simulink model "VB_RIFKF_UWB_INS25"  (R2023a)
settings: Solver=FixedStepAuto  StartTime=0.0  StopTime=500  FixedStep=0.01  RelTol=1e-3
InitFcn:
  | resilient_initNavigation1216;
  | init_param;
  | param_bias;
undefined symbols (not defined in the file or in its folder): dt, g0, gam0_rad, ISUS_flag, lp_GPS_sample_time, lp_Lidar_knoise, lp_Lidar_max, lp_Lidar_min, lp_Lidar_sample_time, lp_Lidar_seed, lp_UWB_knoise, lp_UWB_sample_time, lp_UWB_seed, lp_UWB_XY_max, lp_UWB_XY_min, magnitude, p, P0, P0_RIEKF, param, pd0, pe0, phi0_rad, pn0, psi, psi0_rad, state_dim, vd0, ve0, vn0
libraries: simulink_extras x108, simulink x89, dspstat3 x74, sharedtransform x61, matrix_library x11, sharedTrackingLibrary x8, aerolibconvert2 x5, aerolibtransform2 x5, dspfactors x3
(part 9 of 29)

== system VB_RIFKF_UWB_INS25/No.1_Sensor_Data_Process/Magn_Data_Process ==
  magn_B_guass_ori : Inport
  Data Type Conversion : DataTypeConversion  OutDataTypeStr=single  SaturateOnIntegerOverflow=off  RndMeth=Floor
  MATLAB Function1 : MATLAB Function  Commented=on  TreatAsAtomicUnit=on
  Magn_preprocessing : Subsystem
  MAGN_Data : Outport
  wires:
  magn_B_guass_ori/1 -> Data Type Conversion/1, Magn_preprocessing/1(Magn_B_rad/s_ori)
  Data Type Conversion/1 -> MAGN_Data/1

== system VB_RIFKF_UWB_INS25/No.1_Sensor_Data_Process/Subsystem ==
  Vairspeed : Inport
  Constant : Constant  Value=0  OutDataTypeStr=single
  Mux : Mux  Inputs=3
  TD_baro : Subsystem
  Terminator : Terminator
  VairspeedData : Outport
  wires:
  TD_baro/2(H_baro_TD) -> Mux/1
  Constant/1 -> Mux/3, Mux/2
  Mux/1 -> VairspeedData/1  "VairspeedData"
  Vairspeed/1 -> TD_baro/1(H_baro)
  TD_baro/1(vH_baro_TD) -> Terminator/1  "vH_baro_m/s_TD"

== system VB_RIFKF_UWB_INS25/No.1_Sensor_Data_Process/TOF_Data_Process ==
  TOF_mm_ori : Inport
  QGC_sensor_reinit : Inport  Port=2
  Bus Creator1 : BusCreator  Inputs=4
  Data Type Conversion : DataTypeConversion  OutDataTypeStr=uint8  SaturateOnIntegerOverflow=off  RndMeth=Floor
  Data Type Conversion1 : DataTypeConversion  OutDataTypeStr=single  SaturateOnIntegerOverflow=off  RndMeth=Floor
  Demux : Demux  Outputs=3
  Gain : Gain  Gain=0.01
  Scope : Scope  NumInputPorts=2
  Scope1 : Scope  NumInputPorts=2
  Sum : Sum  Inputs=|-+
  TD_baro : Subsystem
  reinit_TOF : Subsystem
  TOF_Data : Outport
  wires:
  Sum/1 -> Data Type Conversion1/1, Scope1/2  "TOF_Dist_m"
  reinit_TOF/1(dataout) -> Sum/1, Scope1/1
  QGC_sensor_reinit/1 -> reinit_TOF/1(QGC_sensor_reinit)
  Data Type Conversion/1 -> Bus Creator1/4  "TOF_sts"
  Gain/1 -> reinit_TOF/2(Data), Sum/2  "TOF_Dist_m"
  TD_baro/1(vH_TOF_TD) -> Bus Creator1/1, Scope/1  "vH_TOF_m/s_TD"
  Bus Creator1/1 -> TOF_Data/1  "TOF_Data"
  Demux/2 -> Bus Creator1/3  "TOF_Inten"
  TOF_mm_ori/1 -> Demux/1
  Demux/1 -> Gain/1
  Demux/3 -> Data Type Conversion/1  "TOF_sts"
  TD_baro/2(H_TOF_TD) -> Scope/2, Bus Creator1/2  "H_TOF_TD"
  Data Type Conversion1/1 -> TD_baro/1(H_TOF)  "补偿姿态前"

== system VB_RIFKF_UWB_INS25/No.1_Sensor_Data_Process/baro_Data_Process ==
  baro : Inport
  QGC_sensor_reinit : Inport  Port=2
  baro_tem : Inport  Port=3
  Bus Creator : BusCreator  Inputs=2
  Constant : Constant  Value=0  OutDataTypeStr=single
  From Workspace : FromWorkspace  Commented=on  VariableName=[All.t',All.Alt_Ps]
  Gain : Gain  Gain=0.01
  Pressure2Height : Subsystem
  Scope : Scope
  Scope1 : Scope  Commented=on  NumInputPorts=2
  Sum : Sum  Inputs=|+-
  Sum1 : Sum  Commented=on  Inputs=|+-
  Sum2 : Sum  Inputs=|+-
  Switch : Switch  Criteria=u2 > Threshold  Threshold=31  SaturateOnIntegerOverflow=off  InputSameDT=off
  TD_baro : Subsystem
  TemCompensate1 : Subsystem
  reinit_baro0 : Subsystem
  reinit_baro1 : Subsystem  Commented=on
  BARO_Data : Outport  PortDimensions=2
  wires:
  baro_tem/1 -> TemCompensate1/1(baro_tem), Switch/2  "AFCbarotem"
  Pressure2Height/1(H_baro) -> TD_baro/1(H_baro)  "AFC4"
  Switch/1 -> Sum2/2
  baro/1 -> Gain/1  "AFC4"
  Constant/1 -> Switch/1
  TemCompensate1/1(bias) -> Switch/3
  Sum2/1 -> Sum/1, reinit_baro0/2(Data)
  TD_baro/2(H_baro_TD) -> Sum2/1  "H_baro_TD"
  Sum/1 -> Scope1/2, Scope/1, Bus Creator/2  "H_baro_TD"
  reinit_baro0/1(dataout) -> Sum/2
  QGC_sensor_reinit/1 -> reinit_baro1/1(QGC_sensor_reinit), reinit_baro0/1(QGC_sensor_reinit)
  Bus Creator/1 -> BARO_Data/1
  Gain/1 -> Pressure2Height/1(baro)
  TD_baro/1(vH_baro_TD) -> Bus Creator/1  "vH_baro_m/s_TD"
  From Workspace/1 -> reinit_baro1/2(Data), Sum1/1
  reinit_baro1/1(dataout) -> Sum1/2
  Sum1/1 -> Scope1/1

== system VB_RIFKF_UWB_INS25/No.1_Sensor_Data_Process1/GPS_Data_Process ==
  note: GPS_fixtype:
      | 0: 定位不可用或无效
      | 1:单点定位
      | 2:伪距差分
      | 4:RTK固定解
  GPS_Vecef_m/s : Inport
  GPS_LLA_rad : Inport  Port=2
  GPS_fixtype : Inport  Port=3
  hdop_GPS : Inport  Port=4
  QGC_sensor_reinit : Inport  Port=5
  GPS0 : Inport  Port=6
  Bus Creator : BusCreator  Inputs=13
  Demux : Demux  Outputs=3
  Demux1 : Demux  Outputs=3
  Demux3 : Demux  Outputs=3
  GPS_fixtype1 : InportShadow  Port=3
  LLA2NED : Subsystem
  heading_GPS : Subsystem
  GPS_Data : Outport
  wires:
  LLA2NED/1("gpsposNEDout ") -> Demux1/1
  GPS_fixtype1/1 -> LLA2NED/2(GPSfixtype)  "fixtype_gps"
  Bus Creator/1 -> GPS_Data/1
  Demux3/3 -> Bus Creator/3  "H_gps"
  Demux/3 -> Bus Creator/9  "vd_gps"
  Demux/1 -> Bus Creator/7  "vn_gps"
  GPS_LLA_rad/1 -> Demux3/1, LLA2NED/1(gps_LLA_rad)
  Demux/2 -> Bus Creator/8  "ve_gps"
  Demux3/2 -> Bus Creator/2  "lon_gps"
  Demux3/1 -> Bus Creator/1  "lat_gps"
  GPS_fixtype/1 -> Bus Creator/12  "fixtype_gps"
  QGC_sensor_reinit/1 -> LLA2NED/4(QGC_sensor_reinit)  "QGC_sensor_reinit"
  Demux1/1 -> Bus Creator/4  "pos_N_gps"
  Demux1/2 -> Bus Creator/5  "pos_E_gps"
  Demux1/3 -> Bus Creator/6  "pos_D_gps"
  GPS_Vecef_m/s/1 -> LLA2NED/3(GPS_Vecef_m/s)
  LLA2NED/2(gpsvNEDout) -> Demux/1, heading_GPS/1(Vned)
  heading_GPS/1(heading_GPS_rad) -> Bus Creator/10  "heading_GPS_rad"
  heading_GPS/2(heading_GPS_valid) -> Bus Creator/11  "heading_GPS_valid"
  hdop_GPS/1 -> Bus Creator/13  "hdop_GPS"
  GPS0/1 -> LLA2NED/5(GPS0)

== system VB_RIFKF_UWB_INS25/No.1_Sensor_Data_Process1/IMU_Data_Process ==
  gyro_B_rad/s_ori : Inport
  accl_B_m/s_ori : Inport  Port=2
  Bias Eliminate : Subsystem
  Bus Creator : BusCreator  Inputs=2
  accl_preprocessing2 : Subsystem  Commented=on
  gyro_preprocessing2 : Subsystem  Commented=on
  IMU_Data : Outport  PortDimensions=6
  wires:
  Bus Creator/1 -> IMU_Data/1
  accl_B_m/s_ori/1 -> Bus Creator/2  "accl_B_m/s2_LPF"
  Bias Eliminate/1(Out1) -> Bus Creator/1  "gyro_B_rad/s_LPF"
  gyro_B_rad/s_ori/1 -> Bias Eliminate/1(gyro_B_rad/s_ori)  "gyro_B_rad/s_LPF"

== system VB_RIFKF_UWB_INS25/No.1_Sensor_Data_Process1/Magn_Data_Process ==
  magn_B_guass_ori : Inport
  Data Type Conversion : DataTypeConversion  OutDataTypeStr=single  SaturateOnIntegerOverflow=off  RndMeth=Floor
  MATLAB Function1 : MATLAB Function  Commented=on  TreatAsAtomicUnit=on
  Magn_preprocessing : Subsystem
  MAGN_Data : Outport
  wires:
  Data Type Conversion/1 -> MAGN_Data/1
  magn_B_guass_ori/1 -> Magn_preprocessing/1(Magn_B_rad/s_ori), Data Type Conversion/1

== system VB_RIFKF_UWB_INS25/No.1_Sensor_Data_Process1/Subsystem ==
  Vairspeed : Inport
  Constant : Constant  Value=0  OutDataTypeStr=single
  Mux : Mux  Inputs=3
  TD_baro : Subsystem
  Terminator : Terminator
  VairspeedData : Outport
  wires:
  TD_baro/1(vH_baro_TD) -> Terminator/1  "vH_baro_m/s_TD"
  Vairspeed/1 -> TD_baro/1(H_baro)
  Mux/1 -> VairspeedData/1  "VairspeedData"
  Constant/1 -> Mux/2, Mux/3
  TD_baro/2(H_baro_TD) -> Mux/1

== system VB_RIFKF_UWB_INS25/No.1_Sensor_Data_Process1/TOF_Data_Process ==
  TOF_mm_ori : Inport
  QGC_sensor_reinit : Inport  Port=2
  Bus Creator1 : BusCreator  Inputs=4
  Data Type Conversion : DataTypeConversion  OutDataTypeStr=uint8  SaturateOnIntegerOverflow=off  RndMeth=Floor
  Data Type Conversion1 : DataTypeConversion  OutDataTypeStr=single  SaturateOnIntegerOverflow=off  RndMeth=Floor
  Demux : Demux  Outputs=3
  Gain : Gain  Gain=0.01
  Scope : Scope  NumInputPorts=2
  Scope1 : Scope  NumInputPorts=2
  Sum : Sum  Inputs=|-+
  TD_baro : Subsystem
  reinit_TOF : Subsystem
  TOF_Data : Outport
  wires:
  Data Type Conversion1/1 -> TD_baro/1(H_TOF)  "补偿姿态前"
  TD_baro/2(H_TOF_TD) -> Bus Creator1/2, Scope/2  "H_TOF_TD"
  Demux/3 -> Data Type Conversion/1  "TOF_sts"
  Demux/1 -> Gain/1
  TOF_mm_ori/1 -> Demux/1
  Demux/2 -> Bus Creator1/3  "TOF_Inten"
  Bus Creator1/1 -> TOF_Data/1  "TOF_Data"
  TD_baro/1(vH_TOF_TD) -> Scope/1, Bus Creator1/1  "vH_TOF_m/s_TD"
  Gain/1 -> Sum/2, reinit_TOF/2(Data)  "TOF_Dist_m"
  Data Type Conversion/1 -> Bus Creator1/4  "TOF_sts"
  QGC_sensor_reinit/1 -> reinit_TOF/1(QGC_sensor_reinit)
  reinit_TOF/1(dataout) -> Scope1/1, Sum/1
  Sum/1 -> Scope1/2, Data Type Conversion1/1  "TOF_Dist_m"

== system VB_RIFKF_UWB_INS25/No.1_Sensor_Data_Process1/baro_Data_Process ==
  baro : Inport
  QGC_sensor_reinit : Inport  Port=2
  baro_tem : Inport  Port=3
  Bus Creator : BusCreator  Inputs=2
  Constant : Constant  Value=0  OutDataTypeStr=single
  From Workspace : FromWorkspace  Commented=on  VariableName=[All.t',All.Alt_Ps]
  Gain : Gain  Gain=0.01
  Pressure2Height : Subsystem
  Scope : Scope
  Scope1 : Scope  Commented=on  NumInputPorts=2
  Sum : Sum  Inputs=|+-
  Sum1 : Sum  Commented=on  Inputs=|+-
  Sum2 : Sum  Inputs=|+-
  Switch : Switch  Criteria=u2 > Threshold  Threshold=31  SaturateOnIntegerOverflow=off  InputSameDT=off
  TD_baro : Subsystem
  TemCompensate1 : Subsystem
  reinit_baro0 : Subsystem
  reinit_baro1 : Subsystem  Commented=on
  BARO_Data : Outport  PortDimensions=2
  wires:
  Sum1/1 -> Scope1/1
  reinit_baro1/1(dataout) -> Sum1/2
  From Workspace/1 -> Sum1/1, reinit_baro1/2(Data)
  TD_baro/1(vH_baro_TD) -> Bus Creator/1  "vH_baro_m/s_TD"
  Gain/1 -> Pressure2Height/1(baro)
  Bus Creator/1 -> BARO_Data/1
  QGC_sensor_reinit/1 -> reinit_baro0/1(QGC_sensor_reinit), reinit_baro1/1(QGC_sensor_reinit)
  reinit_baro0/1(dataout) -> Sum/2
  Sum/1 -> Bus Creator/2, Scope/1, Scope1/2  "H_baro_TD"
  TD_baro/2(H_baro_TD) -> Sum2/1  "H_baro_TD"
  Sum2/1 -> reinit_baro0/2(Data), Sum/1
  TemCompensate1/1(bias) -> Switch/3
  Constant/1 -> Switch/1
  baro/1 -> Gain/1  "AFC4"
  Switch/1 -> Sum2/2
  Pressure2Height/1(H_baro) -> TD_baro/1(H_baro)  "AFC4"
  baro_tem/1 -> Switch/2, TemCompensate1/1(baro_tem)  "AFCbarotem"

== system VB_RIFKF_UWB_INS25/No.1_Sensor_Data_Process2/GPS_Data_Process ==
  note: GPS_fixtype:
      | 0: 定位不可用或无效
      | 1:单点定位
      | 2:伪距差分
      | 4:RTK固定解
  GPS_Vecef_m/s : Inport
  GPS_LLA_rad : Inport  Port=2
  GPS_fixtype : Inport  Port=3
  hdop_GPS : Inport  Port=4
  QGC_sensor_reinit : Inport  Port=5
  GPS0 : Inport  Port=6
  Bus Creator : BusCreator  Inputs=13
  Demux : Demux  Outputs=3
  Demux1 : Demux  Outputs=3
  Demux3 : Demux  Outputs=3
  GPS_fixtype1 : InportShadow  Port=3
  LLA2NED : Subsystem
  heading_GPS : Subsystem
  GPS_Data : Outport
  wires:
  hdop_GPS/1 -> Bus Creator/13  "hdop_GPS"
  heading_GPS/2(heading_GPS_valid) -> Bus Creator/11  "heading_GPS_valid"
  heading_GPS/1(heading_GPS_rad) -> Bus Creator/10  "heading_GPS_rad"
  LLA2NED/2(gpsvNEDout) -> heading_GPS/1(Vned), Demux/1
  GPS_Vecef_m/s/1 -> LLA2NED/3(GPS_Vecef_m/s)
  Demux1/3 -> Bus Creator/6  "pos_D_gps"
  Demux1/2 -> Bus Creator/5  "pos_E_gps"
  Demux1/1 -> Bus Creator/4  "pos_N_gps"
  QGC_sensor_reinit/1 -> LLA2NED/4(QGC_sensor_reinit)  "QGC_sensor_reinit"
  GPS_fixtype/1 -> Bus Creator/12  "fixtype_gps"
  Demux3/1 -> Bus Creator/1  "lat_gps"
  Demux3/2 -> Bus Creator/2  "lon_gps"
  Demux/2 -> Bus Creator/8  "ve_gps"
  GPS_LLA_rad/1 -> LLA2NED/1(gps_LLA_rad), Demux3/1
  Demux/1 -> Bus Creator/7  "vn_gps"
  Demux/3 -> Bus Creator/9  "vd_gps"
  Demux3/3 -> Bus Creator/3  "H_gps"
  Bus Creator/1 -> GPS_Data/1
  GPS_fixtype1/1 -> LLA2NED/2(GPSfixtype)  "fixtype_gps"
  LLA2NED/1("gpsposNEDout ") -> Demux1/1
  GPS0/1 -> LLA2NED/5(GPS0)

== system VB_RIFKF_UWB_INS25/No.1_Sensor_Data_Process2/IMU_Data_Process ==
  gyro_B_rad/s_ori : Inport
  accl_B_m/s_ori : Inport  Port=2
  Bias Eliminate : Subsystem
  Bus Creator : BusCreator  Inputs=2
  accl_preprocessing2 : Subsystem  Commented=on
  gyro_preprocessing2 : Subsystem  Commented=on
  IMU_Data : Outport  PortDimensions=6
  wires:
  gyro_B_rad/s_ori/1 -> Bias Eliminate/1(gyro_B_rad/s_ori)  "gyro_B_rad/s_LPF"
  Bias Eliminate/1(Out1) -> Bus Creator/1  "gyro_B_rad/s_LPF"
  accl_B_m/s_ori/1 -> Bus Creator/2  "accl_B_m/s2_LPF"
  Bus Creator/1 -> IMU_Data/1

== system VB_RIFKF_UWB_INS25/No.1_Sensor_Data_Process2/Magn_Data_Process ==
  magn_B_guass_ori : Inport
  Data Type Conversion : DataTypeConversion  OutDataTypeStr=single  SaturateOnIntegerOverflow=off  RndMeth=Floor
  MATLAB Function1 : MATLAB Function  Commented=on  TreatAsAtomicUnit=on
  Magn_preprocessing : Subsystem
  MAGN_Data : Outport
  wires:
  magn_B_guass_ori/1 -> Data Type Conversion/1, Magn_preprocessing/1(Magn_B_rad/s_ori)
  Data Type Conversion/1 -> MAGN_Data/1

== system VB_RIFKF_UWB_INS25/No.1_Sensor_Data_Process2/Subsystem ==
  Vairspeed : Inport
  Constant : Constant  Value=0  OutDataTypeStr=single
  Mux : Mux  Inputs=3
  TD_baro : Subsystem
  Terminator : Terminator
  VairspeedData : Outport
  wires:
  TD_baro/2(H_baro_TD) -> Mux/1
  Constant/1 -> Mux/3, Mux/2
  Mux/1 -> VairspeedData/1  "VairspeedData"
  Vairspeed/1 -> TD_baro/1(H_baro)
  TD_baro/1(vH_baro_TD) -> Terminator/1  "vH_baro_m/s_TD"

== system VB_RIFKF_UWB_INS25/No.1_Sensor_Data_Process2/TOF_Data_Process ==
  TOF_mm_ori : Inport
  QGC_sensor_reinit : Inport  Port=2
  Bus Creator1 : BusCreator  Inputs=4
  Data Type Conversion : DataTypeConversion  OutDataTypeStr=uint8  SaturateOnIntegerOverflow=off  RndMeth=Floor
  Data Type Conversion1 : DataTypeConversion  OutDataTypeStr=single  SaturateOnIntegerOverflow=off  RndMeth=Floor
  Demux : Demux  Outputs=3
  Gain : Gain  Gain=0.01
  Scope : Scope  NumInputPorts=2
  Scope1 : Scope  NumInputPorts=2
  Sum : Sum  Inputs=|-+
  TD_baro : Subsystem
  reinit_TOF : Subsystem
  TOF_Data : Outport
  wires:
  Sum/1 -> Data Type Conversion1/1, Scope1/2  "TOF_Dist_m"
  reinit_TOF/1(dataout) -> Sum/1, Scope1/1
  QGC_sensor_reinit/1 -> reinit_TOF/1(QGC_sensor_reinit)
  Data Type Conversion/1 -> Bus Creator1/4  "TOF_sts"
  Gain/1 -> reinit_TOF/2(Data), Sum/2  "TOF_Dist_m"
  TD_baro/1(vH_TOF_TD) -> Bus Creator1/1, Scope/1  "vH_TOF_m/s_TD"
  Bus Creator1/1 -> TOF_Data/1  "TOF_Data"
  Demux/2 -> Bus Creator1/3  "TOF_Inten"
  TOF_mm_ori/1 -> Demux/1
  Demux/1 -> Gain/1
  Demux/3 -> Data Type Conversion/1  "TOF_sts"
  TD_baro/2(H_TOF_TD) -> Scope/2, Bus Creator1/2  "H_TOF_TD"
  Data Type Conversion1/1 -> TD_baro/1(H_TOF)  "补偿姿态前"

== system VB_RIFKF_UWB_INS25/No.1_Sensor_Data_Process2/baro_Data_Process ==
  baro : Inport
  QGC_sensor_reinit : Inport  Port=2
  baro_tem : Inport  Port=3
  Bus Creator : BusCreator  Inputs=2
  Constant : Constant  Value=0  OutDataTypeStr=single
  From Workspace : FromWorkspace  Commented=on  VariableName=[All.t',All.Alt_Ps]
  Gain : Gain  Gain=0.01
  Pressure2Height : Subsystem
  Scope : Scope
  Scope1 : Scope  Commented=on  NumInputPorts=2
  Sum : Sum  Inputs=|+-
  Sum1 : Sum  Commented=on  Inputs=|+-
  Sum2 : Sum  Inputs=|+-
  Switch : Switch  Criteria=u2 > Threshold  Threshold=31  SaturateOnIntegerOverflow=off  InputSameDT=off
  TD_baro : Subsystem
  TemCompensate1 : Subsystem
  reinit_baro0 : Subsystem
  reinit_baro1 : Subsystem  Commented=on
  BARO_Data : Outport  PortDimensions=2
  wires:
  baro_tem/1 -> TemCompensate1/1(baro_tem), Switch/2  "AFCbarotem"
  Pressure2Height/1(H_baro) -> TD_baro/1(H_baro)  "AFC4"
  Switch/1 -> Sum2/2
  baro/1 -> Gain/1  "AFC4"
  Constant/1 -> Switch/1
  TemCompensate1/1(bias) -> Switch/3
  Sum2/1 -> Sum/1, reinit_baro0/2(Data)
  TD_baro/2(H_baro_TD) -> Sum2/1  "H_baro_TD"
  Sum/1 -> Scope1/2, Scope/1, Bus Creator/2  "H_baro_TD"
  reinit_baro0/1(dataout) -> Sum/2
  QGC_sensor_reinit/1 -> reinit_baro1/1(QGC_sensor_reinit), reinit_baro0/1(QGC_sensor_reinit)
  Bus Creator/1 -> BARO_Data/1
  Gain/1 -> Pressure2Height/1(baro)
  TD_baro/1(vH_baro_TD) -> Bus Creator/1  "vH_baro_m/s_TD"
  From Workspace/1 -> reinit_baro1/2(Data), Sum1/1
  reinit_baro1/1(dataout) -> Sum1/2
  Sum1/1 -> Scope1/1

== system VB_RIFKF_UWB_INS25/No.1_Sensor_Data_Process3/GPS_Data_Process ==
  note: GPS_fixtype:
      | 0: 定位不可用或无效
      | 1:单点定位
      | 2:伪距差分
      | 4:RTK固定解
  GPS_Vecef_m/s : Inport
  GPS_LLA_rad : Inport  Port=2
  GPS_fixtype : Inport  Port=3
  hdop_GPS : Inport  Port=4
  QGC_sensor_reinit : Inport  Port=5
  Bus Creator : BusCreator  Inputs=13
  Demux : Demux  Outputs=3
  Demux1 : Demux  Outputs=3
  Demux3 : Demux  Outputs=3
  GPS_fixtype1 : InportShadow  Port=3
  LLA2NED : Subsystem
  heading_GPS : Subsystem
  GPS_Data : Outport
  wires:
  LLA2NED/1("gpsposNEDout ") -> Demux1/1
  GPS_fixtype1/1 -> LLA2NED/2(GPSfixtype)  "fixtype_gps"
  Bus Creator/1 -> GPS_Data/1
  Demux3/3 -> Bus Creator/3  "H_gps"
  Demux/3 -> Bus Creator/9  "vd_gps"
  Demux/1 -> Bus Creator/7  "vn_gps"
  GPS_LLA_rad/1 -> Demux3/1, LLA2NED/1(gps_LLA_rad)
  Demux/2 -> Bus Creator/8  "ve_gps"
  Demux3/2 -> Bus Creator/2  "lon_gps"
  Demux3/1 -> Bus Creator/1  "lat_gps"
  GPS_fixtype/1 -> Bus Creator/12  "fixtype_gps"
  QGC_sensor_reinit/1 -> LLA2NED/4(QGC_sensor_reinit)  "QGC_sensor_reinit"
  Demux1/1 -> Bus Creator/4  "pos_N_gps"
  Demux1/2 -> Bus Creator/5  "pos_E_gps"
  Demux1/3 -> Bus Creator/6  "pos_D_gps"
  GPS_Vecef_m/s/1 -> LLA2NED/3(GPS_Vecef_m/s)
  LLA2NED/2(gpsvNEDout) -> Demux/1, heading_GPS/1(Vned)
  heading_GPS/1(heading_GPS_rad) -> Bus Creator/10  "heading_GPS_rad"
  heading_GPS/2(heading_GPS_valid) -> Bus Creator/11  "heading_GPS_valid"
  hdop_GPS/1 -> Bus Creator/13  "hdop_GPS"

== system VB_RIFKF_UWB_INS25/No.1_Sensor_Data_Process3/IMU_Data_Process ==
  gyro_B_rad/s_ori : Inport
  accl_B_m/s_ori : Inport  Port=2
  Bias Eliminate : Subsystem
  Bus Creator : BusCreator  Inputs=2
  accl_preprocessing2 : Subsystem  Commented=on
  gyro_preprocessing2 : Subsystem  Commented=on
  IMU_Data : Outport  PortDimensions=6
  wires:
  Bus Creator/1 -> IMU_Data/1
  accl_B_m/s_ori/1 -> Bus Creator/2  "accl_B_m/s2_LPF"
  Bias Eliminate/1(Out1) -> Bus Creator/1  "gyro_B_rad/s_LPF"
  gyro_B_rad/s_ori/1 -> Bias Eliminate/1(gyro_B_rad/s_ori)  "gyro_B_rad/s_LPF"

== system VB_RIFKF_UWB_INS25/No.1_Sensor_Data_Process3/Magn_Data_Process ==
  magn_B_guass_ori : Inport
  Data Type Conversion : DataTypeConversion  OutDataTypeStr=single  SaturateOnIntegerOverflow=off  RndMeth=Floor
  MATLAB Function1 : MATLAB Function  Commented=on  TreatAsAtomicUnit=on
  Magn_preprocessing : Subsystem
  MAGN_Data : Outport
  wires:
  Data Type Conversion/1 -> MAGN_Data/1
  magn_B_guass_ori/1 -> Magn_preprocessing/1(Magn_B_rad/s_ori), Data Type Conversion/1

== system VB_RIFKF_UWB_INS25/No.1_Sensor_Data_Process3/Subsystem ==
  Vairspeed : Inport
  Constant : Constant  Value=0  OutDataTypeStr=single
  Mux : Mux  Inputs=3
  TD_baro : Subsystem
  Terminator : Terminator
  VairspeedData : Outport
  wires:
  TD_baro/1(vH_baro_TD) -> Terminator/1  "vH_baro_m/s_TD"
  Vairspeed/1 -> TD_baro/1(H_baro)
  Mux/1 -> VairspeedData/1  "VairspeedData"
  Constant/1 -> Mux/2, Mux/3
  TD_baro/2(H_baro_TD) -> Mux/1

== system VB_RIFKF_UWB_INS25/No.1_Sensor_Data_Process3/TOF_Data_Process ==
  TOF_mm_ori : Inport
  QGC_sensor_reinit : Inport  Port=2
  Bus Creator1 : BusCreator  Inputs=4
  Data Type Conversion : DataTypeConversion  OutDataTypeStr=uint8  SaturateOnIntegerOverflow=off  RndMeth=Floor
  Data Type Conversion1 : DataTypeConversion  OutDataTypeStr=single  SaturateOnIntegerOverflow=off  RndMeth=Floor
  Demux : Demux  Outputs=3
  Gain : Gain  Gain=0.01
  Scope : Scope  NumInputPorts=2
  Scope1 : Scope  NumInputPorts=2
  Sum : Sum  Inputs=|-+
  TD_baro : Subsystem
  reinit_TOF : Subsystem
  TOF_Data : Outport
  wires:
  Data Type Conversion1/1 -> TD_baro/1(H_TOF)  "补偿姿态前"
  TD_baro/2(H_TOF_TD) -> Bus Creator1/2, Scope/2  "H_TOF_TD"
  Demux/3 -> Data Type Conversion/1  "TOF_sts"
  Demux/1 -> Gain/1
  TOF_mm_ori/1 -> Demux/1
  Demux/2 -> Bus Creator1/3  "TOF_Inten"
  Bus Creator1/1 -> TOF_Data/1  "TOF_Data"
  TD_baro/1(vH_TOF_TD) -> Scope/1, Bus Creator1/1  "vH_TOF_m/s_TD"
  Gain/1 -> Sum/2, reinit_TOF/2(Data)  "TOF_Dist_m"
  Data Type Conversion/1 -> Bus Creator1/4  "TOF_sts"
  QGC_sensor_reinit/1 -> reinit_TOF/1(QGC_sensor_reinit)
  reinit_TOF/1(dataout) -> Scope1/1, Sum/1
  Sum/1 -> Scope1/2, Data Type Conversion1/1  "TOF_Dist_m"

== system VB_RIFKF_UWB_INS25/No.1_Sensor_Data_Process3/baro_Data_Process ==
  baro : Inport
  QGC_sensor_reinit : Inport  Port=2
  baro_tem : Inport  Port=3
  Bus Creator : BusCreator  Inputs=2
  Constant : Constant  Value=0  OutDataTypeStr=single
  From Workspace : FromWorkspace  Commented=on  VariableName=[All.t',All.Alt_Ps]
  Gain : Gain  Gain=0.01
  Pressure2Height : Subsystem
  Scope : Scope
  Scope1 : Scope  Commented=on  NumInputPorts=2
  Sum : Sum  Inputs=|+-
  Sum1 : Sum  Commented=on  Inputs=|+-
  Sum2 : Sum  Inputs=|+-
  Switch : Switch  Criteria=u2 > Threshold  Threshold=31  SaturateOnIntegerOverflow=off  InputSameDT=off
  TD_baro : Subsystem
  TemCompensate1 : Subsystem
  reinit_baro0 : Subsystem
  reinit_baro1 : Subsystem  Commented=on
  BARO_Data : Outport  PortDimensions=2
  wires:
  Sum1/1 -> Scope1/1
  reinit_baro1/1(dataout) -> Sum1/2
  From Workspace/1 -> Sum1/1, reinit_baro1/2(Data)
  TD_baro/1(vH_baro_TD) -> Bus Creator/1  "vH_baro_m/s_TD"
  Gain/1 -> Pressure2Height/1(baro)
  Bus Creator/1 -> BARO_Data/1
  QGC_sensor_reinit/1 -> reinit_baro0/1(QGC_sensor_reinit), reinit_baro1/1(QGC_sensor_reinit)
  reinit_baro0/1(dataout) -> Sum/2
  Sum/1 -> Bus Creator/2, Scope/1, Scope1/2  "H_baro_TD"
  TD_baro/2(H_baro_TD) -> Sum2/1  "H_baro_TD"
  Sum2/1 -> reinit_baro0/2(Data), Sum/1
  TemCompensate1/1(bias) -> Switch/3
  Constant/1 -> Switch/1
  baro/1 -> Gain/1  "AFC4"
  Switch/1 -> Sum2/2
  Pressure2Height/1(H_baro) -> TD_baro/1(H_baro)  "AFC4"
  baro_tem/1 -> Switch/2, TemCompensate1/1(baro_tem)  "AFCbarotem"

== system VB_RIFKF_UWB_INS25/No.1_Sensor_Data_Process4/GPS_Data_Process ==
  note: GPS_fixtype:
      | 0: 定位不可用或无效
      | 1:单点定位
      | 2:伪距差分
      | 4:RTK固定解
  GPS_Vecef_m/s : Inport
  GPS_LLA_rad : Inport  Port=2
  GPS_fixtype : Inport  Port=3
  hdop_GPS : Inport  Port=4
  QGC_sensor_reinit : Inport  Port=5
  Bus Creator : BusCreator  Inputs=13
  Demux : Demux  Outputs=3
  Demux1 : Demux  Outputs=3
  Demux3 : Demux  Outputs=3
  GPS_fixtype1 : InportShadow  Port=3
  LLA2NED : Subsystem
  heading_GPS : Subsystem
  GPS_Data : Outport
  GPS0 : Outport  Port=2
  GPS_noerr : Outport  Port=3
  wires:
  LLA2NED/4(gpsposNED_noerr) -> GPS_noerr/1
  LLA2NED/3(GPS0) -> GPS0/1
  LLA2NED/1("gpsposNEDout ") -> Demux1/1
  GPS_fixtype1/1 -> LLA2NED/2(GPSfixtype)  "fixtype_gps"
  Bus Creator/1 -> GPS_Data/1
  Demux3/3 -> Bus Creator/3  "H_gps"
  Demux/3 -> Bus Creator/9  "vd_gps"
  Demux/1 -> Bus Creator/7  "vn_gps"
  GPS_LLA_rad/1 -> Demux3/1, LLA2NED/1(gps_LLA_rad)
  Demux/2 -> Bus Creator/8  "ve_gps"
  Demux3/2 -> Bus Creator/2  "lon_gps"
  Demux3/1 -> Bus Creator/1  "lat_gps"
  GPS_fixtype/1 -> Bus Creator/12  "fixtype_gps"
  QGC_sensor_reinit/1 -> LLA2NED/4(QGC_sensor_reinit)  "QGC_sensor_reinit"
  Demux1/1 -> Bus Creator/4  "pos_N_gps"
  Demux1/2 -> Bus Creator/5  "pos_E_gps"
  Demux1/3 -> Bus Creator/6  "pos_D_gps"
  GPS_Vecef_m/s/1 -> LLA2NED/3(GPS_Vecef_m/s)
  LLA2NED/2(gpsvNEDout) -> Demux/1, heading_GPS/1(Vned)
  heading_GPS/1(heading_GPS_rad) -> Bus Creator/10  "heading_GPS_rad"
  heading_GPS/2(heading_GPS_valid) -> Bus Creator/11  "heading_GPS_valid"
  hdop_GPS/1 -> Bus Creator/13  "hdop_GPS"

== system VB_RIFKF_UWB_INS25/No.1_Sensor_Data_Process4/IMU_Data_Process ==
  gyro_B_rad/s_ori : Inport
  accl_B_m/s_ori : Inport  Port=2
  Bias Eliminate : Subsystem
  Bus Creator : BusCreator  Inputs=2
  accl_preprocessing2 : Subsystem  Commented=on
  gyro_preprocessing2 : Subsystem  Commented=on
  IMU_Data : Outport  PortDimensions=6
  wires:
  Bus Creator/1 -> IMU_Data/1
  accl_B_m/s_ori/1 -> Bus Creator/2  "accl_B_m/s2_LPF"
  Bias Eliminate/1(Out1) -> Bus Creator/1  "gyro_B_rad/s_LPF"
  gyro_B_rad/s_ori/1 -> Bias Eliminate/1(gyro_B_rad/s_ori)  "gyro_B_rad/s_LPF"

== system VB_RIFKF_UWB_INS25/No.1_Sensor_Data_Process4/Magn_Data_Process ==
  magn_B_guass_ori : Inport
  Data Type Conversion : DataTypeConversion  OutDataTypeStr=single  SaturateOnIntegerOverflow=off  RndMeth=Floor
  MATLAB Function1 : MATLAB Function  Commented=on  TreatAsAtomicUnit=on
  Magn_preprocessing : Subsystem
  MAGN_Data : Outport
  wires:
  Data Type Conversion/1 -> MAGN_Data/1
  magn_B_guass_ori/1 -> Magn_preprocessing/1(Magn_B_rad/s_ori), Data Type Conversion/1

== system VB_RIFKF_UWB_INS25/No.1_Sensor_Data_Process4/Subsystem ==
  Vairspeed : Inport
  Constant : Constant  Value=0  OutDataTypeStr=single
  Mux : Mux  Inputs=3
  TD_baro : Subsystem
  Terminator : Terminator
  VairspeedData : Outport
  wires:
  TD_baro/1(vH_baro_TD) -> Terminator/1  "vH_baro_m/s_TD"
  Vairspeed/1 -> TD_baro/1(H_baro)
  Mux/1 -> VairspeedData/1  "VairspeedData"
  Constant/1 -> Mux/2, Mux/3
  TD_baro/2(H_baro_TD) -> Mux/1

== system VB_RIFKF_UWB_INS25/No.1_Sensor_Data_Process4/TOF_Data_Process ==
  TOF_mm_ori : Inport
  QGC_sensor_reinit : Inport  Port=2
  Bus Creator1 : BusCreator  Inputs=4
  Data Type Conversion : DataTypeConversion  OutDataTypeStr=uint8  SaturateOnIntegerOverflow=off  RndMeth=Floor
  Data Type Conversion1 : DataTypeConversion  OutDataTypeStr=single  SaturateOnIntegerOverflow=off  RndMeth=Floor
  Demux : Demux  Outputs=3
  Gain : Gain  Gain=0.01
  Scope : Scope  NumInputPorts=2
  Scope1 : Scope  NumInputPorts=2
  Sum : Sum  Inputs=|-+
  TD_baro : Subsystem
  reinit_TOF : Subsystem
  TOF_Data : Outport
  wires:
  Data Type Conversion1/1 -> TD_baro/1(H_TOF)  "补偿姿态前"
  TD_baro/2(H_TOF_TD) -> Bus Creator1/2, Scope/2  "H_TOF_TD"
  Demux/3 -> Data Type Conversion/1  "TOF_sts"
  Demux/1 -> Gain/1
  TOF_mm_ori/1 -> Demux/1
  Demux/2 -> Bus Creator1/3  "TOF_Inten"
  Bus Creator1/1 -> TOF_Data/1  "TOF_Data"
  TD_baro/1(vH_TOF_TD) -> Scope/1, Bus Creator1/1  "vH_TOF_m/s_TD"
  Gain/1 -> Sum/2, reinit_TOF/2(Data)  "TOF_Dist_m"
  Data Type Conversion/1 -> Bus Creator1/4  "TOF_sts"
  QGC_sensor_reinit/1 -> reinit_TOF/1(QGC_sensor_reinit)
  reinit_TOF/1(dataout) -> Scope1/1, Sum/1
  Sum/1 -> Scope1/2, Data Type Conversion1/1  "TOF_Dist_m"

== system VB_RIFKF_UWB_INS25/No.1_Sensor_Data_Process4/baro_Data_Process ==
  baro : Inport
  QGC_sensor_reinit : Inport  Port=2
  baro_tem : Inport  Port=3
  Bus Creator : BusCreator  Inputs=2
  Constant : Constant  Value=0  OutDataTypeStr=single
  From Workspace : FromWorkspace  Commented=on  VariableName=[All.t',All.Alt_Ps]
  Gain : Gain  Gain=0.01
  Pressure2Height : Subsystem
  Scope : Scope
  Scope1 : Scope  Commented=on  NumInputPorts=2
  Sum : Sum  Inputs=|+-
  Sum1 : Sum  Commented=on  Inputs=|+-
  Sum2 : Sum  Inputs=|+-
  Switch : Switch  Criteria=u2 > Threshold  Threshold=31  SaturateOnIntegerOverflow=off  InputSameDT=off
  TD_baro : Subsystem
  TemCompensate1 : Subsystem
  reinit_baro0 : Subsystem
  reinit_baro1 : Subsystem  Commented=on
  BARO_Data : Outport  PortDimensions=2
  wires:
  Sum1/1 -> Scope1/1
  reinit_baro1/1(dataout) -> Sum1/2
  From Workspace/1 -> Sum1/1, reinit_baro1/2(Data)
  TD_baro/1(vH_baro_TD) -> Bus Creator/1  "vH_baro_m/s_TD"
  Gain/1 -> Pressure2Height/1(baro)
  Bus Creator/1 -> BARO_Data/1
  QGC_sensor_reinit/1 -> reinit_baro0/1(QGC_sensor_reinit), reinit_baro1/1(QGC_sensor_reinit)
  reinit_baro0/1(dataout) -> Sum/2
  Sum/1 -> Bus Creator/2, Scope/1, Scope1/2  "H_baro_TD"
  TD_baro/2(H_baro_TD) -> Sum2/1  "H_baro_TD"
  Sum2/1 -> reinit_baro0/2(Data), Sum/1
  TemCompensate1/1(bias) -> Switch/3
  Constant/1 -> Switch/1
  baro/1 -> Gain/1  "AFC4"
  Switch/1 -> Sum2/2
  Pressure2Height/1(H_baro) -> TD_baro/1(H_baro)  "AFC4"
  baro_tem/1 -> Switch/2, TemCompensate1/1(baro_tem)  "AFCbarotem"

== system VB_RIFKF_UWB_INS25/read FC1_hf/Subsystem ==
  u : Inport
  MATLAB Function : MATLAB Function  TreatAsAtomicUnit=on
  Memory : Memory
  y : Outport
  wires:
  Memory/1 -> MATLAB Function/2(u_1)
  MATLAB Function/1(y) -> y/1, Memory/1
  u/1 -> MATLAB Function/1(u)

== system VB_RIFKF_UWB_INS25/read FC1_hf/Subsystem1 ==
  u : Inport
  MATLAB Function : MATLAB Function  TreatAsAtomicUnit=on
  Memory : Memory
  y : Outport
  wires:
  u/1 -> MATLAB Function/1(u)
  MATLAB Function/1(y) -> Memory/1, y/1
  Memory/1 -> MATLAB Function/2(u_1)

== system VB_RIFKF_UWB_INS25/read FC1_hf/Subsystem2 ==
  u : Inport
  MATLAB Function : MATLAB Function  TreatAsAtomicUnit=on
  Memory : Memory
  y : Outport
  wires:
  Memory/1 -> MATLAB Function/2(u_1)
  MATLAB Function/1(y) -> y/1, Memory/1
  u/1 -> MATLAB Function/1(u)

== system VB_RIFKF_UWB_INS25/read FC1_hf/Subsystem3 ==
  u : Inport
  MATLAB Function : MATLAB Function  TreatAsAtomicUnit=on
  Memory : Memory
  y : Outport
  wires:
  u/1 -> MATLAB Function/1(u)
  MATLAB Function/1(y) -> Memory/1, y/1
  Memory/1 -> MATLAB Function/2(u_1)

== system VB_RIFKF_UWB_INS25/read FC1_hf/Subsystem4 ==
  u : Inport
  MATLAB Function : MATLAB Function  TreatAsAtomicUnit=on
  Memory : Memory
  y : Outport
  wires:
  Memory/1 -> MATLAB Function/2(u_1)
  MATLAB Function/1(y) -> y/1, Memory/1
  u/1 -> MATLAB Function/1(u)

== system VB_RIFKF_UWB_INS25/read FC1_hf/Subsystem5 ==
  u : Inport
  MATLAB Function : MATLAB Function  TreatAsAtomicUnit=on
  Memory : Memory
  y : Outport
  wires:
  u/1 -> MATLAB Function/1(u)
  MATLAB Function/1(y) -> Memory/1, y/1
  Memory/1 -> MATLAB Function/2(u_1)

== system VB_RIFKF_UWB_INS25/read FC1_hf/Subsystem6 ==
  u : Inport
  MATLAB Function : MATLAB Function  TreatAsAtomicUnit=on
  Memory : Memory
  y : Outport
  wires:
  Memory/1 -> MATLAB Function/2(u_1)
  MATLAB Function/1(y) -> y/1, Memory/1
  u/1 -> MATLAB Function/1(u)

== system VB_RIFKF_UWB_INS25/read FC1_hf/Subsystem7 ==
  u : Inport
  MATLAB Function : MATLAB Function  TreatAsAtomicUnit=on
  Memory : Memory
  y : Outport
  wires:
  u/1 -> MATLAB Function/1(u)
  MATLAB Function/1(y) -> Memory/1, y/1
  Memory/1 -> MATLAB Function/2(u_1)

== system VB_RIFKF_UWB_INS25/read FC1_hf/Subsystem8 ==
  u : Inport
  MATLAB Function : MATLAB Function  TreatAsAtomicUnit=on
  Memory : Memory
  y : Outport
  wires:
  Memory/1 -> MATLAB Function/2(u_1)
  MATLAB Function/1(y) -> y/1, Memory/1
  u/1 -> MATLAB Function/1(u)

== system VB_RIFKF_UWB_INS25/read FC1_zy/Subsystem ==
  u : Inport
  MATLAB Function : MATLAB Function  TreatAsAtomicUnit=on
  Memory : Memory
  y : Outport
  wires:
  Memory/1 -> MATLAB Function/2(u_1)
  MATLAB Function/1(y) -> y/1, Memory/1
  u/1 -> MATLAB Function/1(u)

== system VB_RIFKF_UWB_INS25/read FC1_zy/Subsystem1 ==
  u : Inport
  MATLAB Function : MATLAB Function  TreatAsAtomicUnit=on
  Memory : Memory
  y : Outport
  wires:
  u/1 -> MATLAB Function/1(u)
  MATLAB Function/1(y) -> Memory/1, y/1
  Memory/1 -> MATLAB Function/2(u_1)

== system VB_RIFKF_UWB_INS25/read FC1_zy/Subsystem2 ==
  u : Inport
  MATLAB Function : MATLAB Function  TreatAsAtomicUnit=on
  Memory : Memory
  y : Outport
  wires:
  Memory/1 -> MATLAB Function/2(u_1)
  MATLAB Function/1(y) -> y/1, Memory/1
  u/1 -> MATLAB Function/1(u)

== system VB_RIFKF_UWB_INS25/read FC6_zy2/Subsystem ==
  u : Inport
  MATLAB Function : MATLAB Function  TreatAsAtomicUnit=on
  Memory : Memory
  y : Outport
  wires:
  Memory/1 -> MATLAB Function/2(u_1)
  MATLAB Function/1(y) -> y/1, Memory/1
  u/1 -> MATLAB Function/1(u)

== system VB_RIFKF_UWB_INS25/read FC6_zy2/Subsystem1 ==
  u : Inport
  MATLAB Function : MATLAB Function  TreatAsAtomicUnit=on
  Memory : Memory
  y : Outport
  wires:
  u/1 -> MATLAB Function/1(u)
  MATLAB Function/1(y) -> Memory/1, y/1
  Memory/1 -> MATLAB Function/2(u_1)

== system VB_RIFKF_UWB_INS25/read FC6_zy2/Subsystem2 ==
  u : Inport
  MATLAB Function : MATLAB Function  TreatAsAtomicUnit=on
  Memory : Memory
  y : Outport
  wires:
  Memory/1 -> MATLAB Function/2(u_1)
  MATLAB Function/1(y) -> y/1, Memory/1
  u/1 -> MATLAB Function/1(u)

== system VB_RIFKF_UWB_INS25/相对传感器模拟1/Subsystem ==
  "psi " : Inport
  laser model : Subsystem
  psi  out : Outport
  wires:
  "psi "/1 -> laser model/1(psi & theta)
  laser model/1(psi out) -> psi  out/1

== system VB_RIFKF_UWB_INS25/相对传感器模拟1/Subsystem2 ==
  r_xyz : Inport
  radar model : Subsystem
  r_xyz out : Outport
  wires:
  r_xyz/1 -> radar model/1(r_xyz)
  radar model/1(r_xyz out) -> r_xyz out/1

== system VB_RIFKF_UWB_INS25/相对传感器模拟2/Subsystem ==
  "psi " : Inport
  laser model : Subsystem
  psi  out : Outport
  wires:
  laser model/1(psi out) -> psi  out/1
  "psi "/1 -> laser model/1(psi & theta)

== system VB_RIFKF_UWB_INS25/相对传感器模拟2/Subsystem2 ==
  r_xyz : Inport
  radar model : Subsystem
  r_xyz out : Outport
  wires:
  radar model/1(r_xyz out) -> r_xyz out/1
  r_xyz/1 -> radar model/1(r_xyz)

== system VB_RIFKF_UWB_INS25/相对传感器模拟3/Subsystem ==
  "psi " : Inport
  laser model : Subsystem
  psi  out : Outport
  wires:
  laser model/1(psi out) -> psi  out/1
  "psi "/1 -> laser model/1(psi & theta)

== system VB_RIFKF_UWB_INS25/相对传感器模拟3/Subsystem2 ==
  r_xyz : Inport
  radar model : Subsystem
  r_xyz out : Outport
  wires:
  radar model/1(r_xyz out) -> r_xyz out/1
  r_xyz/1 -> radar model/1(r_xyz)

== system VB_RIFKF_UWB_INS25/相对传感器模拟4/Subsystem ==
  "psi " : Inport
  laser model : Subsystem
  psi  out : Outport
  wires:
  "psi "/1 -> laser model/1(psi & theta)
  laser model/1(psi out) -> psi  out/1

== system VB_RIFKF_UWB_INS25/相对传感器模拟4/Subsystem2 ==
  r_xyz : Inport
  radar model : Subsystem
  r_xyz out : Outport
  wires:
  r_xyz/1 -> radar model/1(r_xyz)
  radar model/1(r_xyz out) -> r_xyz out/1

== system VB_RIFKF_UWB_INS25/ER EKF M1/Bus_Constructor2/Rotation_output ==
  RotationData : Inport
  Bus Creator : BusCreator  Inputs=4
  Bus Selector3 : BusSelector  OutputSignals=DCM_b_n
  Data Type Conversion1 : DataTypeConversion  OutDataTypeStr=single  SaturateOnIntegerOverflow=off  RndMeth=Floor
  Data Type Conversion11 : DataTypeConversion  OutDataTypeStr=single  SaturateOnIntegerOverflow=off  RndMeth=Floor
  Data Type Conversion12 : DataTypeConversion  OutDataTypeStr=double  SaturateOnIntegerOverflow=off  RndMeth=Floor
  Demux : Demux  Outputs=3
  Direction Cosine Matrix to Rotation Angles : sharedtransform/Direction Cosine Matrix to Rotation Angles  rotationOrder=ZYX  aMode=aMode  action=None  tolerance=eps(2)
      settings: LibrarySourceBlock=|
      | aerolibtransform2/Direction Cosine Matrix
      | to Rotation Angles
  Direction Cosine Matrix to Quaternions : sharedtransform/Direction Cosine Matrix  to Quaternions  aMode=0  action=None  tolerance=eps(2)
      settings: LibrarySourceBlock=|
      | aerolibtransform2/Direction Cosine Matrix
      | to Quaternions
  Radians to Degrees : simulink_extras/Transformations/Radians to Degrees
  Scope : Scope
  Signal Copy1 : SignalConversion  OverrideOpt=off
  Transpose : Math  Operator=transpose
  psi_theta_phi_rad : Outport
  wires:
  Direction Cosine Matrix to Quaternions/1 -> Data Type Conversion1/1  "q"
  Radians to Degrees/1 -> Data Type Conversion11/1
  Transpose/1 -> Data Type Conversion12/1
  Data Type Conversion12/1 -> Direction Cosine Matrix to Quaternions/1, Direction Cosine Matrix to Rotation Angles/1
  RotationData/1 -> Signal Copy1/1
  Signal Copy1/1 -> Bus Selector3/1
  Bus Selector3/1 -> Transpose/1  "<DCM_b_n>"
  Direction Cosine Matrix to Rotation Angles/1 -> Radians to Degrees/1  "psi_theta_phi"
  Bus Creator/1 -> psi_theta_phi_rad/1
  Demux/1 -> Bus Creator/1  "psi_rad"
  Demux/2 -> Bus Creator/2  "theta_rad"
  Demux/3 -> Bus Creator/3  "phi_rad"
  Data Type Conversion11/1 -> Scope/1, Demux/1  "ER EKF"
  Data Type Conversion1/1 -> Bus Creator/4  "q"

== system VB_RIFKF_UWB_INS25/ER EKF M1/Error State Kalman Filter/Cal Q1 ==
  Constant : Constant  Value=dt  OutDataTypeStr=double
  MATLAB Function1 : MATLAB Function  TreatAsAtomicUnit=on
  Qd : Outport
  wires:
  MATLAB Function1/1(Q) -> Qd/1
  Constant/1 -> MATLAB Function1/1(dt)

== system VB_RIFKF_UWB_INS25/ER EKF M1/Error State Kalman Filter/Extended Kalman Filter1 ==
  Q : Inport
  Enable1 : Inport  Port=2
  y1 : Inport  Port=3
  R1 : Inport  Port=4
  BlockOrdering : Constant  Value=true()  OutDataTypeStr=boolean
  Correct1 : Subsystem  AncestorBlock=sharedTrackingLibrary/Extras/EKFCorrect  TreatAsAtomicUnit=on  SystemSampleTime=p.SampleTimes.MeasurementFcn(1)  mask(EKFCorrect){ProcessedMaskData=p}
      mask init:
      | if strcmp(get_param(bdroot,'SimulationStatus'),'stopped')
      |     pM = [];
      |     SampleTime = [];
      |     DataType = [];
      |     SLFcnsToRegister = {};
      | else
      |     [pM,SampleTime] = ...
      |         matlabshared.tracking.internal.blocks.maskInitializationFcnEKFCorrector...
      |         (gcbh, ProcessedMaskData);
      |     [DataType,SLFcnsToRegister] = ...
      |         matlabshared.tracking.internal.blocks.maskInitializationFcnRegisterSLFcn(ProcessedMaskData, pM);
      | end
      settings: LibrarySourceBlock=sharedTrackingLibrary/Extras/EKFCorrect
  DataStoreMemory - P : DataStoreMemory  DataStoreName=P  InitialValue=p.InitialCovariance  ShowAdditionalParam=off  OutDataTypeStr=p.DataType
  DataStoreMemory - x : DataStoreMemory  DataStoreName=x  InitialValue=p.InitialState  ShowAdditionalParam=off  OutDataTypeStr=p.DataType
  DataTypeConversion_Enable1 : DataTypeConversion  OutDataTypeStr=boolean  SaturateOnIntegerOverflow=off  RndMeth=Floor
  DataTypeConversion_Q : DataTypeConversion  OutDataTypeStr=p.DataType  SaturateOnIntegerOverflow=off  RndMeth=Floor
  DataTypeConversion_R1 : DataTypeConversion  OutDataTypeStr=p.DataType  SaturateOnIntegerOverflow=off  RndMeth=Floor
  DataTypeConversion_uMeas1 : DataTypeConversion  OutDataTypeStr=p.DataType  SaturateOnIntegerOverflow=off  RndMeth=Floor
  DataTypeConversion_uState : DataTypeConversion  OutDataTypeStr=p.DataType  SaturateOnIntegerOverflow=off  RndMeth=Floor
  DataTypeConversion_y1 : DataTypeConversion  OutDataTypeStr=p.DataType  SaturateOnIntegerOverflow=off  RndMeth=Floor
  MeasurementFcn1Inputs : Constant  Value=0  OutDataTypeStr=p.DataType  SampleTime=p.SampleTimes.MeasurementFcn(1)
  Output : Subsystem  TreatAsAtomicUnit=on  SystemSampleTime=p.SampleTimes.Output
  Predict : Subsystem  TreatAsAtomicUnit=on  SystemSampleTime=p.SampleTimes.StateTransitionFcn  mask(EKFPredict){ProcessedMaskData=p}
      mask init:
      | if strcmp(get_param(bdroot,'SimulationStatus'),'stopped')
      |     pS = [];
      |     SampleTime = [];
      |     DataType = [];
      |     SLFcnsToRegister = {};
      | else
      |     [pS,SampleTime] = ...
      |         matlabshared.tracking.internal.blocks.maskInitializationFcnEKFPredictor(ProcessedMaskData);
      |     [DataType,SLFcnsToRegister] = ...
      |         matlabshared.tracking.internal.blocks.maskInitializationFcnRegisterSLFcn(ProcessedMaskData, pS);
      | end
  StateTransitionFcnInputs : Constant  Value=0  OutDataTypeStr=p.DataType  SampleTime=p.SampleTimes.StateTransitionFcn
  checkMeasurementFcn1Signals : S-Function  FunctionName=ekfukfCheckSignals  Parameters=signalCheck.BlockPath, signalCheck.MeasurementFcn{1}.PortNames, signalCheck.MeasurementFcn{1}.SampleTime, signalCheck.DataType, signalCheck.MeasurementFcn{1}.PortDimensions, 1, signalCheck.MeasurementFcn{1}.HasAdditiveNoise  SFunctionDeploymentMode=off  EnableBusSupport=off
  checkStateTransitionFcnSignals : S-Function  FunctionName=ekfukfCheckSignals  Parameters=signalCheck.BlockPath, signalCheck.StateTransitionFcn.PortNames, signalCheck.StateTransitionFcn.SampleTime, signalCheck.DataType, signalCheck.StateTransitionFcn.PortDimensions, 0, signalCheck.StateTransitionFcn.HasAdditiveNoise  SFunctionDeploymentMode=off  EnableBusSupport=off
  xhat : Outport  VectorParamsAs1DForOutWhenUnconnected=off
  P : Outport  Port=2
  wires:
  y1/1 -> checkMeasurementFcn1Signals/2, DataTypeConversion_y1/1
  R1/1 -> checkMeasurementFcn1Signals/3, DataTypeConversion_R1/1
  Q/1 -> checkStateTransitionFcnSignals/1, DataTypeConversion_Q/1
  DataTypeConversion_Q/1 -> Predict/1(Q)
  Enable1/1 -> checkMeasurementFcn1Signals/1, DataTypeConversion_Enable1/1
  DataTypeConversion_Enable1/1 -> Correct1/Enable
  Output/2(P) -> P/1
  Output/1(x) -> xhat/1
  StateTransitionFcnInputs/1 -> checkStateTransitionFcnSignals/2, DataTypeConversion_uState/1
  DataTypeConversion_uState/1 -> Predict/2(uState)
  DataTypeConversion_y1/1 -> Correct1/1(yMeas)
  MeasurementFcn1Inputs/1 -> checkMeasurementFcn1Signals/4, DataTypeConversion_uMeas1/1
  DataTypeConversion_R1/1 -> Correct1/2(R)
  DataTypeConversion_uMeas1/1 -> Correct1/3(uMeas)
  BlockOrdering/1 -> [FirstOperation]
  [FirstOperation] -> Correct1/4(uBlockOrdering)
  [AfterCorrect] -> Output/1(uBlockOrdering)
  Output/3(yBlockOrdering) -> [AfterOutput]
  [AfterOutput] -> Predict/3(uBlockOrdering)
  Correct1/1(yBlockOrdering) -> [AfterCorrect]

== system VB_RIFKF_UWB_INS25/ER EKF M1/Error State Kalman Filter/Simulink Function - GPS Measurements ==
  GPSMeasurementFcn : TriggerPort  TriggerType=function-call  IsSimulinkFunction=on  FunctionName=GPSMeasurementFcn  FunctionVisibility=scoped  VariantControl=Variant
  Add : Sum
  Constant6 : Constant  Value=[eye(6),zeros(6,9)]  OutDataTypeStr=single
  Display : Display
  Product : Product  Multiplication=Matrix(*)
  x : ArgIn  DisableCoverage=on  OutDataTypeStr=single  PortDimensions=15  ArgumentName=x
  v : ArgIn  DisableCoverage=on  Port=2  OutDataTypeStr=single  PortDimensions=6  ArgumentName=v
  y : ArgOut  DisableCoverage=on  OutDataTypeStr=single  PortDimensions=6  ArgumentName=y
  wires:
  Add/1 -> y/1
  Product/1 -> Add/1
  x/1 -> Product/2
  Constant6/1 -> Display/1, Product/1
  v/1 -> Add/2

== system VB_RIFKF_UWB_INS25/ER EKF M1/Error State Kalman Filter/Simulink Function - GPS Measurements1 ==
  DCM_b_n : Inport
  DynamicMeasurementFcn_Dyn : TriggerPort  TriggerType=function-call  IsSimulinkFunction=on  FunctionName=DynamicMeasurementFcn_Dyn  FunctionVisibility=scoped  VariantControl=Variant
  Add : Sum  Commented=on
  Add1 : Sum
  Constant : Constant  Commented=on  Value=dt  OutDataTypeStr=single
  Constant6 : Constant  Value=[zeros(3,3),eye(3),zeros(3,12);zeros(3,15),eye(3)]  OutDataTypeStr=single
  Data Type Conversion6 : DataTypeConversion  Commented=on  OutDataTypeStr=single  SaturateOnIntegerOverflow=off  RndMeth=Floor
  From7 : From  Commented=on  GotoTag=DCM_b_n
  Goto : Goto  Commented=on  GotoTag=DCM_b_n
  MATLAB Function1 : MATLAB Function  Commented=on  TreatAsAtomicUnit=on
  Product : Product  Commented=on  Multiplication=Matrix(*)
  Product1 : Product  Multiplication=Matrix(*)
  x : ArgIn  DisableCoverage=on  OutDataTypeStr=single  PortDimensions=18  ArgumentName=x
  v : ArgIn  DisableCoverage=on  Port=2  OutDataTypeStr=single  PortDimensions=6  ArgumentName=v
  y : ArgOut  DisableCoverage=on  OutDataTypeStr=single  PortDimensions=6  ArgumentName=y
  wires:
  x/1 -> Product1/2
  Constant6/1 -> Product1/1
  Product1/1 -> Add1/1
  v/1 -> Add1/2
  Add1/1 -> y/1
  Data Type Conversion6/1 -> Product/1
  DCM_b_n/1 -> Goto/1
  Constant/1 -> MATLAB Function1/2(dt)
  From7/1 -> MATLAB Function1/1(Cbn)
  MATLAB Function1/1(H) -> Data Type Conversion6/1
  Product/1 -> Add/1

== system VB_RIFKF_UWB_INS25/ER EKF M1/Error State Kalman Filter/Simulink Function - GPS Measurements2 ==
  ZUPTMeasurementFcn2 : TriggerPort  TriggerType=function-call  IsSimulinkFunction=on  FunctionName=ZUPTMeasurementFcn2  FunctionVisibility=scoped  VariantControl=Variant
  Add : Sum
  Constant6 : Constant  Value=[zeros(3,3),eye(3),zeros(3,12)]  OutDataTypeStr=single
  Product : Product  Multiplication=Matrix(*)
  x : ArgIn  DisableCoverage=on  OutDataTypeStr=single  PortDimensions=18  ArgumentName=x
  v : ArgIn  DisableCoverage=on  Port=2  OutDataTypeStr=single  PortDimensions=3  ArgumentName=v
  y : ArgOut  DisableCoverage=on  OutDataTypeStr=single  PortDimensions=3  ArgumentName=y
  wires:
  v/1 -> Add/2
  Constant6/1 -> Product/1
  x/1 -> Product/2
  Product/1 -> Add/1
  Add/1 -> y/1

== system VB_RIFKF_UWB_INS25/ER EKF M1/Error State Kalman Filter/Simulink Function - GPS Measurements4 ==
  psi12 : Inport
  psi13 : Inport  Port=2
  p2 : Inport  Port=3
  p3 : Inport  Port=4
  p_INS : Inport  Port=5
  UWBMeasurementFcn_Dyn : TriggerPort  TriggerType=function-call  IsSimulinkFunction=on  FunctionName=UWBMeasurementFcn_Dyn  VariantControl=Variant
  Add : Sum
  Constant6 : Constant  Commented=on  Value=[zeros(3,3),eye(3),zeros(3,12)]  OutDataTypeStr=single
  Delay : Delay  DelayLength=1
  Display : Display
  MATLAB Function1 : MATLAB Function  TreatAsAtomicUnit=on
  MATLAB Function2 : MATLAB Function  TreatAsAtomicUnit=on
  Product : Product  Multiplication=Matrix(*)
  Scope : Scope
  x : ArgIn  DisableCoverage=on  OutDataTypeStr=single  PortDimensions=15  ArgumentName=x
  v : ArgIn  DisableCoverage=on  Port=2  OutDataTypeStr=single  PortDimensions=6  ArgumentName=v
  y : ArgOut  DisableCoverage=on  OutDataTypeStr=single  PortDimensions=6  ArgumentName=y
  wires:
  p_INS/1 -> Delay/1, MATLAB Function1/3(p_INS)
  p3/1 -> MATLAB Function1/2(p3)
  p2/1 -> MATLAB Function1/1(p2)
  MATLAB Function1/1(H) -> Scope/1, Product/1, Display/1
  psi13/1 -> MATLAB Function2/2(psi13)
  psi12/1 -> MATLAB Function2/1(psi12)
  v/1 -> Add/2
  Constant6/1 -> ?
  x/1 -> Product/2
  Product/1 -> Add/1
  Add/1 -> y/1
  Delay/1 -> MATLAB Function1/4(p_INS_k_1)

== system VB_RIFKF_UWB_INS25/ER EKF M1/Error State Kalman Filter/Simulink Function - State Transition ==
  DCM_b_n : Inport
  wxyz : Inport  Port=2
  fbxyz : Inport  Port=3
  stateTransitionFcn : TriggerPort  TriggerType=function-call  IsSimulinkFunction=on  FunctionName=stateTransitionFcn  FunctionVisibility=scoped  VariantControl=Variant
  Add : Sum
  Cal Phi : Subsystem
  Constant : Constant  Value=0.01  OutDataTypeStr=single
  Data Type Conversion1 : DataTypeConversion  OutDataTypeStr=single  SaturateOnIntegerOverflow=off  RndMeth=Floor
  Data Type Conversion6 : DataTypeConversion  OutDataTypeStr=single  SaturateOnIntegerOverflow=off  RndMeth=Floor
  MATLAB Function : MATLAB Function  TreatAsAtomicUnit=on
  Product1 : Product  Multiplication=Matrix(*)
  Product2 : Product  Multiplication=Matrix(*)
  Transpose : Math  Operator=transpose
  x : ArgIn  DisableCoverage=on  OutDataTypeStr=single  PortDimensions=15  ArgumentName=x
  w : ArgIn  Port=2  OutDataTypeStr=single  PortDimensions=12  ArgumentName=w
  xNext : ArgOut  DisableCoverage=on  OutDataTypeStr=single  PortDimensions=15  ArgumentName=xNext
  wires:
  Data Type Conversion6/1 -> Add/2
  Data Type Conversion1/1 -> Add/1
  Cal Phi/1(Phi) -> Product2/1
  fbxyz/1 -> [fbxyz]
  wxyz/1 -> [wxyz]
  DCM_b_n/1 -> [DCM_b_n]
  Constant/1 -> MATLAB Function/3(dt)
  [wxyz] -> MATLAB Function/2(wxyz)
  Transpose/1 -> MATLAB Function/1(Cnb)
  [DCM_b_n] -> Transpose/1
  [DCM_b_n] -> Cal Phi/1(<DCM_b_n>)
  [wxyz] -> Cal Phi/2(wxyz)
  [fbxyz] -> Cal Phi/3(axyz)
  Add/1 -> xNext/1
  Product1/1 -> Data Type Conversion1/1
  w/1 -> Product1/2
  MATLAB Function/1(G) -> Product1/1
  Product2/1 -> Data Type Conversion6/1
  x/1 -> Product2/2

== system VB_RIFKF_UWB_INS25/ER EKF M1/Error State Kalman Filter/Simulink Function - State Transition Jacobian ==
  DCM_b_n : Inport
  wxyz : Inport  Port=2
  fbxyz : Inport  Port=3
  stateTransitionJacobianFcn : TriggerPort  TriggerType=function-call  IsSimulinkFunction=on  FunctionName=stateTransitionJacobianFcn  FunctionVisibility=scoped  VariantControl=Variant
  Cal Phi1 : Subsystem
  Constant : Constant  Value=0.01  OutDataTypeStr=single
  Data Type Conversion1 : DataTypeConversion  OutDataTypeStr=single  SaturateOnIntegerOverflow=off  RndMeth=Floor
  Data Type Conversion6 : DataTypeConversion  OutDataTypeStr=single  SaturateOnIntegerOverflow=off  RndMeth=Floor
  MATLAB Function : MATLAB Function  TreatAsAtomicUnit=on
  Terminator : Terminator
  Terminator1 : Terminator
  Transpose : Math  Operator=transpose
  x : ArgIn  DisableCoverage=on  OutDataTypeStr=single  PortDimensions=15  ArgumentName=x
  w : ArgIn  Port=2  OutDataTypeStr=single  PortDimensions=12  ArgumentName=w
  A : ArgOut  DisableCoverage=on  OutDataTypeStr=single  PortDimensions=[15 15]  ArgumentName=A
  G : ArgOut  Port=2  OutDataTypeStr=single  PortDimensions=[15 12]  ArgumentName=G
  wires:
  Data Type Conversion1/1 -> G/1
  Data Type Conversion6/1 -> A/1
  Constant/1 -> MATLAB Function/3(dt)
  Transpose/1 -> MATLAB Function/1(Cnb)
  [DCM_b_n] -> Transpose/1
  [wxyz] -> MATLAB Function/2(wxyz)
  [DCM_b_n] -> Cal Phi1/1(<DCM_b_n>)
  [fbxyz] -> Cal Phi1/3(axyz)
  [wxyz] -> Cal Phi1/2(wxyz)
  wxyz/1 -> [wxyz]
  fbxyz/1 -> [fbxyz]
  DCM_b_n/1 -> [DCM_b_n]
  Cal Phi1/1(Phi) -> Data Type Conversion6/1
  w/1 -> Terminator1/1
  x/1 -> Terminator/1
  MATLAB Function/1(G) -> Data Type Conversion1/1

== system VB_RIFKF_UWB_INS25/ER EKF M1/Error State Kalman Filter/Subsystem ==
  data : Inport
  Detect Change : simulink/Logic and Bit Operations/Detect Change  vinit=0  InputProcessing=Columns as channels (frame based)  OutDataTypeStr=boolean
  Detect Change1 : simulink/Logic and Bit Operations/Detect Change  vinit=0  InputProcessing=Columns as channels (frame based)  OutDataTypeStr=boolean
  From Workspace2 : FromWorkspace  VariableName=[time(1:(end-1)),FCS1.data_hf_st.lat(1:(end-1))]
  From Workspace7 : FromWorkspace  Commented=on  VariableName=[All.t',All.vn]
  Selector : Selector  InputPortWidth=3  IndexOptions=Index vector (dialog)  Indices=[3]  OutputSizes=1
  Zero-Order Hold : ZeroOrderHold  SampleTime=0.2
  Zero-Order Hold1 : ZeroOrderHold  SampleTime=0.01
  flag : Outport
  wires:
  Zero-Order Hold/1 -> Selector/1
  data/1 -> Zero-Order Hold/1
  Selector/1 -> Zero-Order Hold1/1
  Detect Change1/1 -> flag/1
  Zero-Order Hold1/1 -> Detect Change/1
  From Workspace2/1 -> Detect Change1/1  "lat"
